simulink model "TST_PTCOP_TrqCnv"  (R2016b)
settings: Solver=FixedStepDiscrete  StartTime=0.0  StopTime=simTime  FixedStep=sampleTime  RelTol=1e-3
values from neighbouring files (symbols this model uses):
  testCase = 1    [initTST_PTCOP_TrqCnv_001.m]
libraries: simulink x8, UnitTest_Lib x6
settings Model: Creator=zhengjinyan  LastModifiedBy=zhengjinyan
settings DebuggingCC: SignalRangeChecking=error

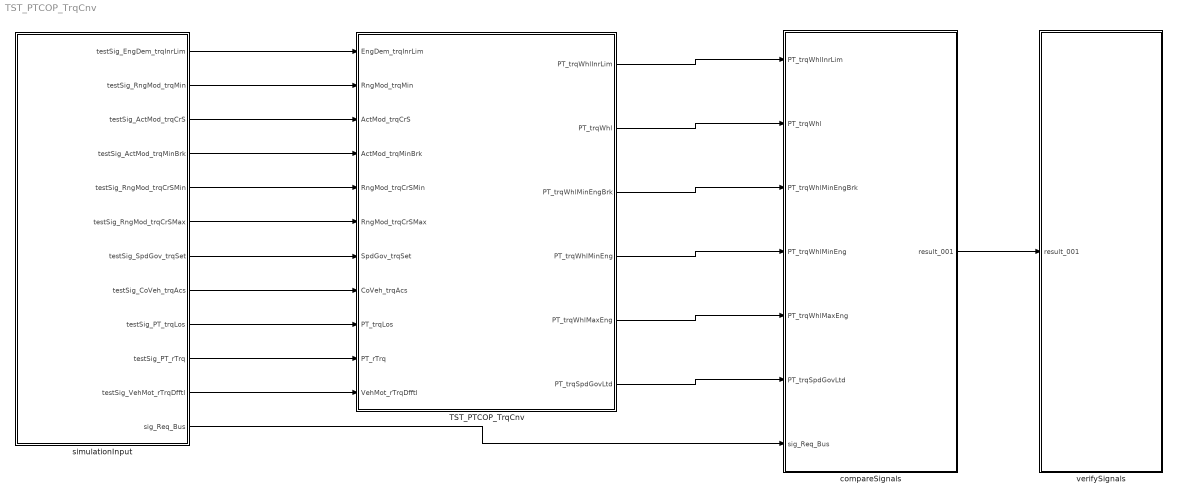
== system TST_PTCOP_TrqCnv ==
  TST_PTCOP_TrqCnv : Subsystem
  compareSignals : Subsystem
  simulationInput : Subsystem
  verifySignals : Subsystem
  wires:
  simulationInput/1(testSig_EngDem_trqInrLim) -> TST_PTCOP_TrqCnv/1(EngDem_trqInrLim)
  simulationInput/2(testSig_RngMod_trqMin) -> TST_PTCOP_TrqCnv/2(RngMod_trqMin)
  simulationInput/3(testSig_ActMod_trqCrS) -> TST_PTCOP_TrqCnv/3(ActMod_trqCrS)
  simulationInput/4(testSig_ActMod_trqMinBrk) -> TST_PTCOP_TrqCnv/4(ActMod_trqMinBrk)
  simulationInput/5(testSig_RngMod_trqCrSMin) -> TST_PTCOP_TrqCnv/5(RngMod_trqCrSMin)
  simulationInput/6(testSig_RngMod_trqCrSMax) -> TST_PTCOP_TrqCnv/6(RngMod_trqCrSMax)
  simulationInput/7(testSig_SpdGov_trqSet) -> TST_PTCOP_TrqCnv/7(SpdGov_trqSet)
  simulationInput/8(testSig_CoVeh_trqAcs) -> TST_PTCOP_TrqCnv/8(CoVeh_trqAcs)
  simulationInput/9(testSig_PT_trqLos) -> TST_PTCOP_TrqCnv/9(PT_trqLos)
  simulationInput/10(testSig_PT_rTrq) -> TST_PTCOP_TrqCnv/10(PT_rTrq)
  simulationInput/11(testSig_VehMot_rTrqDfftl) -> TST_PTCOP_TrqCnv/11(VehMot_rTrqDfftl)
  TST_PTCOP_TrqCnv/1(PT_trqWhlInrLim) -> compareSignals/1(PT_trqWhlInrLim)
  TST_PTCOP_TrqCnv/2(PT_trqWhl) -> compareSignals/2(PT_trqWhl)
  TST_PTCOP_TrqCnv/3(PT_trqWhlMinEngBrk) -> compareSignals/3(PT_trqWhlMinEngBrk)
  TST_PTCOP_TrqCnv/4(PT_trqWhlMinEng) -> compareSignals/4(PT_trqWhlMinEng)
  TST_PTCOP_TrqCnv/5(PT_trqWhlMaxEng) -> compareSignals/5(PT_trqWhlMaxEng)
  TST_PTCOP_TrqCnv/6(PT_trqSpdGovLtd) -> compareSignals/6(PT_trqSpdGovLtd)
  simulationInput/12(sig_Req_Bus) -> compareSignals/7(sig_Req_Bus)
  compareSignals/1(result_001) -> verifySignals/1(result_001)

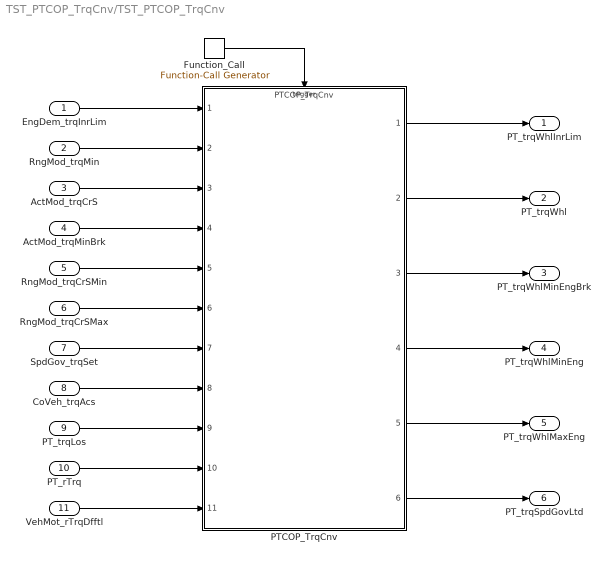
== system TST_PTCOP_TrqCnv/TST_PTCOP_TrqCnv ==
  EngDem_trqInrLim : Inport
  RngMod_trqMin : Inport  Port=2
  ActMod_trqCrS : Inport  Port=3
  ActMod_trqMinBrk : Inport  Port=4
  RngMod_trqCrSMin : Inport  Port=5
  RngMod_trqCrSMax : Inport  Port=6
  SpdGov_trqSet : Inport  Port=7
  CoVeh_trqAcs : Inport  Port=8
  PT_trqLos : Inport  Port=9
  PT_rTrq : Inport  Port=10
  VehMot_rTrqDfftl : Inport  Port=11
  Function_Call : simulink/Ports & Subsystems/Function-Call Generator  sample_time=sampleTime  numberOfIterations=1
  PTCOP_TrqCnv : ModelReference  ModelNameDialog=PTCOP_TrqCnv  SimulationMode=Normal  ModelReferenceVersion=1.5  TriggerPortName=function  TriggerPortTriggerType=function-call  TriggerPortStatesWhenEnabling=held
  PT_trqWhlInrLim : Outport
  PT_trqWhl : Outport  Port=2
  PT_trqWhlMinEngBrk : Outport  Port=3
  PT_trqWhlMinEng : Outport  Port=4
  PT_trqWhlMaxEng : Outport  Port=5
  PT_trqSpdGovLtd : Outport  Port=6
  wires:
  Function_Call/1 -> PTCOP_TrqCnv/Trigger
  EngDem_trqInrLim/1 -> PTCOP_TrqCnv/1
  RngMod_trqMin/1 -> PTCOP_TrqCnv/2
  ActMod_trqCrS/1 -> PTCOP_TrqCnv/3
  ActMod_trqMinBrk/1 -> PTCOP_TrqCnv/4
  RngMod_trqCrSMin/1 -> PTCOP_TrqCnv/5
  RngMod_trqCrSMax/1 -> PTCOP_TrqCnv/6
  SpdGov_trqSet/1 -> PTCOP_TrqCnv/7
  CoVeh_trqAcs/1 -> PTCOP_TrqCnv/8
  PT_trqLos/1 -> PTCOP_TrqCnv/9
  PT_rTrq/1 -> PTCOP_TrqCnv/10
  VehMot_rTrqDfftl/1 -> PTCOP_TrqCnv/11
  PTCOP_TrqCnv/1 -> PT_trqWhlInrLim/1
  PTCOP_TrqCnv/2 -> PT_trqWhl/1
  PTCOP_TrqCnv/3 -> PT_trqWhlMinEngBrk/1
  PTCOP_TrqCnv/4 -> PT_trqWhlMinEng/1
  PTCOP_TrqCnv/5 -> PT_trqWhlMaxEng/1
  PTCOP_TrqCnv/6 -> PT_trqSpdGovLtd/1

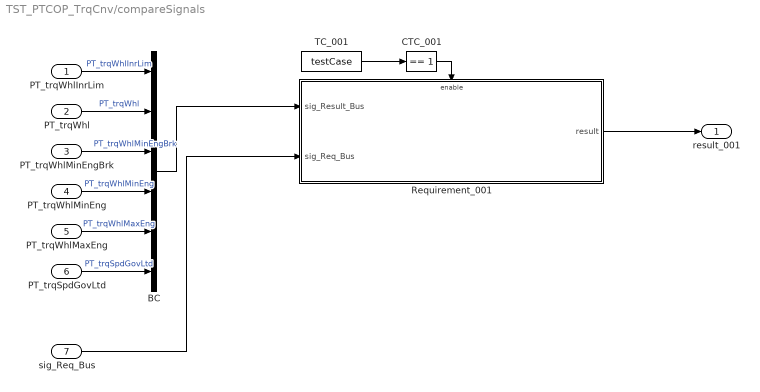
== system TST_PTCOP_TrqCnv/compareSignals ==
  PT_trqWhlInrLim : Inport
  PT_trqWhl : Inport  Port=2
  PT_trqWhlMinEngBrk : Inport  Port=3
  PT_trqWhlMinEng : Inport  Port=4
  PT_trqWhlMaxEng : Inport  Port=5
  PT_trqSpdGovLtd : Inport  Port=6
  sig_Req_Bus : Inport  Port=7
  BC : BusCreator  Inputs=6
  CTC_001 : simulink/Logic and Bit Operations/Compare To Constant  relop===  const=1  OutDataTypeStr=boolean
  Requirement_001 : Subsystem
  TC_001 : Constant  Value=testCase
  result_001 : Outport
  wires:
  PT_trqWhlInrLim/1 -> BC/1  "PT_trqWhlInrLim"
  PT_trqWhl/1 -> BC/2  "PT_trqWhl"
  PT_trqWhlMinEngBrk/1 -> BC/3  "PT_trqWhlMinEngBrk"
  PT_trqWhlMinEng/1 -> BC/4  "PT_trqWhlMinEng"
  PT_trqWhlMaxEng/1 -> BC/5  "PT_trqWhlMaxEng"
  PT_trqSpdGovLtd/1 -> BC/6  "PT_trqSpdGovLtd"
  TC_001/1 -> CTC_001/1
  CTC_001/1 -> Requirement_001/Enable
  sig_Req_Bus/1 -> Requirement_001/2(sig_Req_Bus)
  BC/1 -> Requirement_001/1(sig_Result_Bus)
  Requirement_001/1(result) -> result_001/1

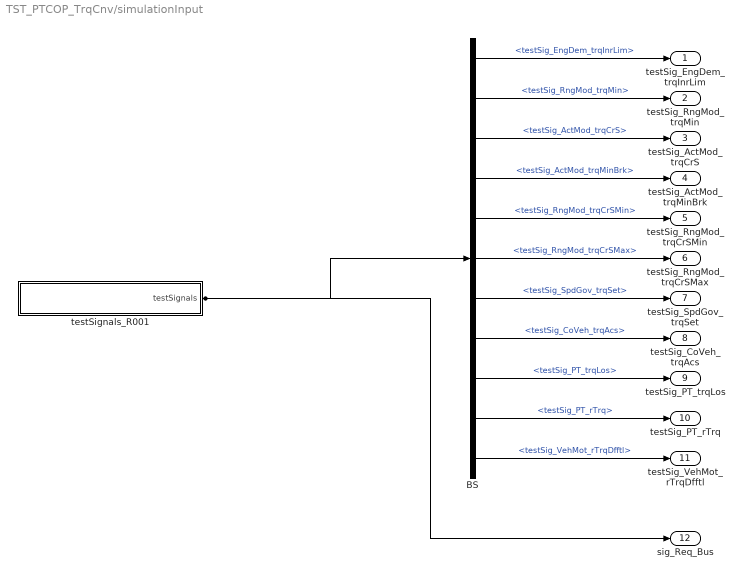
== system TST_PTCOP_TrqCnv/simulationInput ==
  BS : BusSelector  OutputSignals=testSig_EngDem_trqInrLim,testSig_RngMod_trqMin,testSig_ActMod_trqCrS,testSig_ActMod_trqMinBrk,testSig_RngMod_trqCrSMin,testSig_RngMod_trqCrSMax,testSig_SpdGov_trqSet,testSig_CoVeh_trqAcs,testSig_PT_trqLos,testSig_PT_rTrq,testSig_VehMot_rTrqDfftl
  testSignals_R001 : Subsystem
  testSig_EngDem_trqInrLim : Outport
  testSig_RngMod_trqMin : Outport  Port=2
  testSig_ActMod_trqCrS : Outport  Port=3
  testSig_ActMod_trqMinBrk : Outport  Port=4
  testSig_RngMod_trqCrSMin : Outport  Port=5
  testSig_RngMod_trqCrSMax : Outport  Port=6
  testSig_SpdGov_trqSet : Outport  Port=7
  testSig_CoVeh_trqAcs : Outport  Port=8
  testSig_PT_trqLos : Outport  Port=9
  testSig_PT_rTrq : Outport  Port=10
  testSig_VehMot_rTrqDfftl : Outport  Port=11
  sig_Req_Bus : Outport  Port=12
  wires:
  BS/1 -> testSig_EngDem_trqInrLim/1  "<testSig_EngDem_trqInrLim>"
  BS/2 -> testSig_RngMod_trqMin/1  "<testSig_RngMod_trqMin>"
  BS/3 -> testSig_ActMod_trqCrS/1  "<testSig_ActMod_trqCrS>"
  BS/4 -> testSig_ActMod_trqMinBrk/1  "<testSig_ActMod_trqMinBrk>"
  BS/5 -> testSig_RngMod_trqCrSMin/1  "<testSig_RngMod_trqCrSMin>"
  BS/6 -> testSig_RngMod_trqCrSMax/1  "<testSig_RngMod_trqCrSMax>"
  BS/7 -> testSig_SpdGov_trqSet/1  "<testSig_SpdGov_trqSet>"
  BS/8 -> testSig_CoVeh_trqAcs/1  "<testSig_CoVeh_trqAcs>"
  BS/9 -> testSig_PT_trqLos/1  "<testSig_PT_trqLos>"
  BS/10 -> testSig_PT_rTrq/1  "<testSig_PT_rTrq>"
  BS/11 -> testSig_VehMot_rTrqDfftl/1  "<testSig_VehMot_rTrqDfftl>"
  testSignals_R001/1(testSignals) -> BS/1, sig_Req_Bus/1

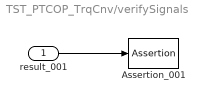
== system TST_PTCOP_TrqCnv/verifySignals ==
  result_001 : Inport
  Assertion_001 : Assertion  Enabled=off
  wires:
  result_001/1 -> Assertion_001/1

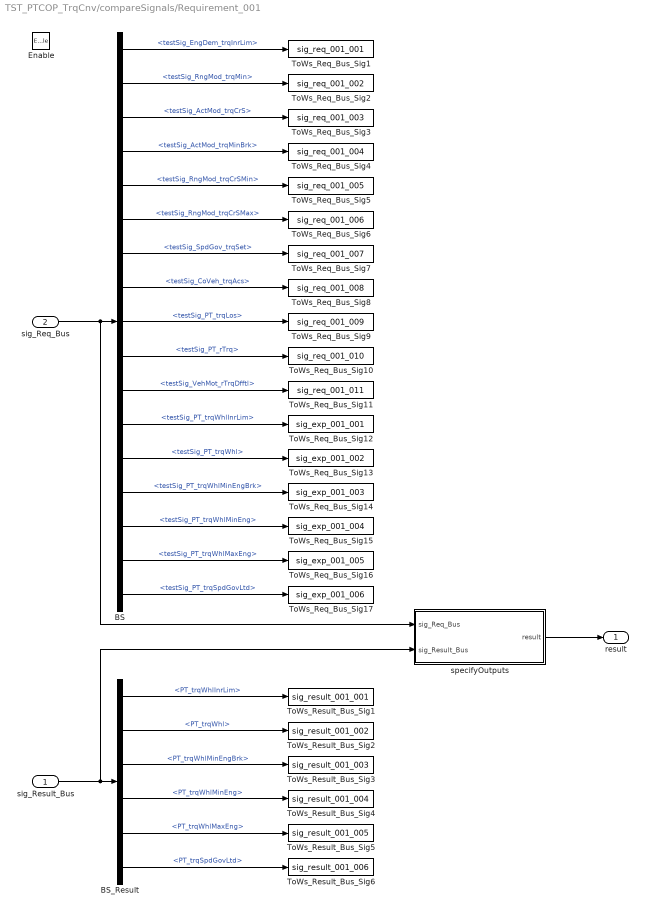
== system TST_PTCOP_TrqCnv/compareSignals/Requirement_001 ==
  sig_Result_Bus : Inport
  sig_Req_Bus : Inport  Port=2
  Enable : EnablePort
  BS : BusSelector  OutputSignals=testSig_EngDem_trqInrLim,testSig_RngMod_trqMin,testSig_ActMod_trqCrS,testSig_ActMod_trqMinBrk,testSig_RngMod_trqCrSMin,testSig_RngMod_trqCrSMax,testSig_SpdGov_trqSet,testSig_CoVeh_trqAcs,testSig_PT_trqLos,testSig_PT_rTrq,testSig_VehMot_rTrqDfftl,testSig_PT_trqWhlInrLim,testSig_PT_trqWhl,testSig_PT_trqWhlMinEngBrk,testSig_PT_trqWhlMinEng,testSig_PT_trqWhlMaxEng,testSig_PT_trqSpdGovLtd
  BS_Result : BusSelector  OutputSignals=PT_trqWhlInrLim,PT_trqWhl,PT_trqWhlMinEngBrk,PT_trqWhlMinEng,PT_trqWhlMaxEng,PT_trqSpdGovLtd
  ToWs_Req_Bus_Sig1 : ToWorkspace  VariableName=sig_req_001_001  SaveFormat=Structure With Time
  ToWs_Req_Bus_Sig10 : ToWorkspace  VariableName=sig_req_001_010  SaveFormat=Structure With Time
  ToWs_Req_Bus_Sig11 : ToWorkspace  VariableName=sig_req_001_011  SaveFormat=Structure With Time
  ToWs_Req_Bus_Sig12 : ToWorkspace  VariableName=sig_exp_001_001  SaveFormat=Structure With Time
  ToWs_Req_Bus_Sig13 : ToWorkspace  VariableName=sig_exp_001_002  SaveFormat=Structure With Time
  ToWs_Req_Bus_Sig14 : ToWorkspace  VariableName=sig_exp_001_003  SaveFormat=Structure With Time
  ToWs_Req_Bus_Sig15 : ToWorkspace  VariableName=sig_exp_001_004  SaveFormat=Structure With Time
  ToWs_Req_Bus_Sig16 : ToWorkspace  VariableName=sig_exp_001_005  SaveFormat=Structure With Time
  ToWs_Req_Bus_Sig17 : ToWorkspace  VariableName=sig_exp_001_006  SaveFormat=Structure With Time
  ToWs_Req_Bus_Sig2 : ToWorkspace  VariableName=sig_req_001_002  SaveFormat=Structure With Time
  ToWs_Req_Bus_Sig3 : ToWorkspace  VariableName=sig_req_001_003  SaveFormat=Structure With Time
  ToWs_Req_Bus_Sig4 : ToWorkspace  VariableName=sig_req_001_004  SaveFormat=Structure With Time
  ToWs_Req_Bus_Sig5 : ToWorkspace  VariableName=sig_req_001_005  SaveFormat=Structure With Time
  ToWs_Req_Bus_Sig6 : ToWorkspace  VariableName=sig_req_001_006  SaveFormat=Structure With Time
  ToWs_Req_Bus_Sig7 : ToWorkspace  VariableName=sig_req_001_007  SaveFormat=Structure With Time
  ToWs_Req_Bus_Sig8 : ToWorkspace  VariableName=sig_req_001_008  SaveFormat=Structure With Time
  ToWs_Req_Bus_Sig9 : ToWorkspace  VariableName=sig_req_001_009  SaveFormat=Structure With Time
  ToWs_Result_Bus_Sig1 : ToWorkspace  VariableName=sig_result_001_001  SaveFormat=Structure With Time
  ToWs_Result_Bus_Sig2 : ToWorkspace  VariableName=sig_result_001_002  SaveFormat=Structure With Time
  ToWs_Result_Bus_Sig3 : ToWorkspace  VariableName=sig_result_001_003  SaveFormat=Structure With Time
  ToWs_Result_Bus_Sig4 : ToWorkspace  VariableName=sig_result_001_004  SaveFormat=Structure With Time
  ToWs_Result_Bus_Sig5 : ToWorkspace  VariableName=sig_result_001_005  SaveFormat=Structure With Time
  ToWs_Result_Bus_Sig6 : ToWorkspace  VariableName=sig_result_001_006  SaveFormat=Structure With Time
  specifyOutputs : Subsystem
  result : Outport
  wires:
  sig_Req_Bus/1 -> BS/1, specifyOutputs/1(sig_Req_Bus)
  BS/1 -> ToWs_Req_Bus_Sig1/1  "<testSig_EngDem_trqInrLim>"
  BS/2 -> ToWs_Req_Bus_Sig2/1  "<testSig_RngMod_trqMin>"
  BS/3 -> ToWs_Req_Bus_Sig3/1  "<testSig_ActMod_trqCrS>"
  BS/4 -> ToWs_Req_Bus_Sig4/1  "<testSig_ActMod_trqMinBrk>"
  BS/5 -> ToWs_Req_Bus_Sig5/1  "<testSig_RngMod_trqCrSMin>"
  BS/6 -> ToWs_Req_Bus_Sig6/1  "<testSig_RngMod_trqCrSMax>"
  BS/7 -> ToWs_Req_Bus_Sig7/1  "<testSig_SpdGov_trqSet>"
  BS/8 -> ToWs_Req_Bus_Sig8/1  "<testSig_CoVeh_trqAcs>"
  BS/9 -> ToWs_Req_Bus_Sig9/1  "<testSig_PT_trqLos>"
  BS/10 -> ToWs_Req_Bus_Sig10/1  "<testSig_PT_rTrq>"
  BS/11 -> ToWs_Req_Bus_Sig11/1  "<testSig_VehMot_rTrqDfftl>"
  BS/12 -> ToWs_Req_Bus_Sig12/1  "<testSig_PT_trqWhlInrLim>"
  BS/13 -> ToWs_Req_Bus_Sig13/1  "<testSig_PT_trqWhl>"
  BS/14 -> ToWs_Req_Bus_Sig14/1  "<testSig_PT_trqWhlMinEngBrk>"
  BS/15 -> ToWs_Req_Bus_Sig15/1  "<testSig_PT_trqWhlMinEng>"
  BS/16 -> ToWs_Req_Bus_Sig16/1  "<testSig_PT_trqWhlMaxEng>"
  BS/17 -> ToWs_Req_Bus_Sig17/1  "<testSig_PT_trqSpdGovLtd>"
  sig_Result_Bus/1 -> BS_Result/1, specifyOutputs/2(sig_Result_Bus)
  BS_Result/1 -> ToWs_Result_Bus_Sig1/1  "<PT_trqWhlInrLim>"
  BS_Result/2 -> ToWs_Result_Bus_Sig2/1  "<PT_trqWhl>"
  BS_Result/3 -> ToWs_Result_Bus_Sig3/1  "<PT_trqWhlMinEngBrk>"
  BS_Result/4 -> ToWs_Result_Bus_Sig4/1  "<PT_trqWhlMinEng>"
  BS_Result/5 -> ToWs_Result_Bus_Sig5/1  "<PT_trqWhlMaxEng>"
  BS_Result/6 -> ToWs_Result_Bus_Sig6/1  "<PT_trqSpdGovLtd>"
  specifyOutputs/1(result) -> result/1

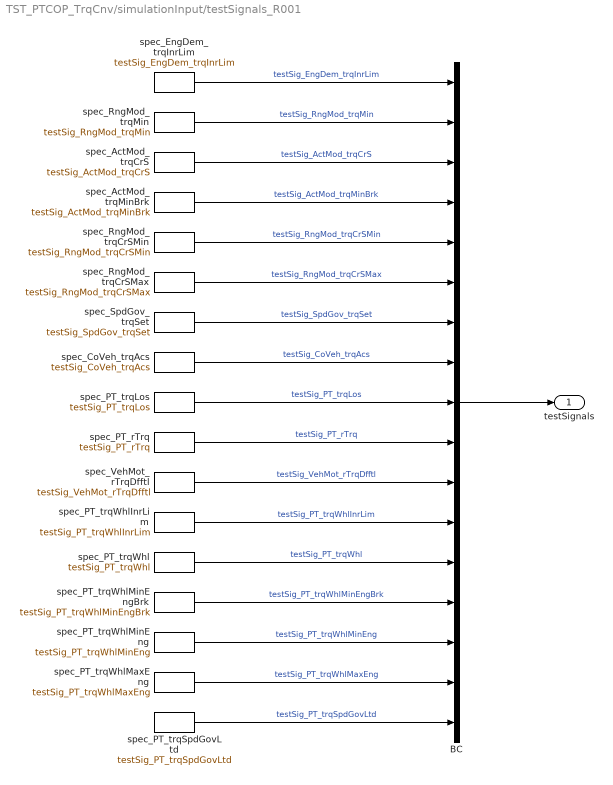
== system TST_PTCOP_TrqCnv/simulationInput/testSignals_R001 ==
  BC : BusCreator  Inputs=17
  spec_ActMod_trqCrS : FromWorkspace  VariableName=testSig_ActMod_trqCrS  Interpolate=off  OutputAfterFinalValue=Holding final value
  spec_ActMod_trqMinBrk : FromWorkspace  VariableName=testSig_ActMod_trqMinBrk  Interpolate=off  OutputAfterFinalValue=Holding final value
  spec_CoVeh_trqAcs : FromWorkspace  VariableName=testSig_CoVeh_trqAcs  Interpolate=off  OutputAfterFinalValue=Holding final value
  spec_EngDem_trqInrLim : FromWorkspace  VariableName=testSig_EngDem_trqInrLim  Interpolate=off  OutputAfterFinalValue=Holding final value
  spec_PT_rTrq : FromWorkspace  VariableName=testSig_PT_rTrq  Interpolate=off  OutputAfterFinalValue=Holding final value
  spec_PT_trqLos : FromWorkspace  VariableName=testSig_PT_trqLos  Interpolate=off  OutputAfterFinalValue=Holding final value
  spec_PT_trqSpdGovLtd : FromWorkspace  VariableName=testSig_PT_trqSpdGovLtd  Interpolate=off  OutputAfterFinalValue=Holding final value
  spec_PT_trqWhl : FromWorkspace  VariableName=testSig_PT_trqWhl  Interpolate=off  OutputAfterFinalValue=Holding final value
  spec_PT_trqWhlInrLim : FromWorkspace  VariableName=testSig_PT_trqWhlInrLim  Interpolate=off  OutputAfterFinalValue=Holding final value
  spec_PT_trqWhlMaxEng : FromWorkspace  VariableName=testSig_PT_trqWhlMaxEng  Interpolate=off  OutputAfterFinalValue=Holding final value
  spec_PT_trqWhlMinEng : FromWorkspace  VariableName=testSig_PT_trqWhlMinEng  Interpolate=off  OutputAfterFinalValue=Holding final value
  spec_PT_trqWhlMinEngBrk : FromWorkspace  VariableName=testSig_PT_trqWhlMinEngBrk  Interpolate=off  OutputAfterFinalValue=Holding final value
  spec_RngMod_trqCrSMax : FromWorkspace  VariableName=testSig_RngMod_trqCrSMax  Interpolate=off  OutputAfterFinalValue=Holding final value
  spec_RngMod_trqCrSMin : FromWorkspace  VariableName=testSig_RngMod_trqCrSMin  Interpolate=off  OutputAfterFinalValue=Holding final value
  spec_RngMod_trqMin : FromWorkspace  VariableName=testSig_RngMod_trqMin  Interpolate=off  OutputAfterFinalValue=Holding final value
  spec_SpdGov_trqSet : FromWorkspace  VariableName=testSig_SpdGov_trqSet  Interpolate=off  OutputAfterFinalValue=Holding final value
  spec_VehMot_rTrqDfftl : FromWorkspace  VariableName=testSig_VehMot_rTrqDfftl  Interpolate=off  OutputAfterFinalValue=Holding final value
  testSignals : Outport
  wires:
  BC/1 -> testSignals/1
  spec_EngDem_trqInrLim/1 -> BC/1  "testSig_EngDem_trqInrLim"
  spec_RngMod_trqMin/1 -> BC/2  "testSig_RngMod_trqMin"
  spec_ActMod_trqCrS/1 -> BC/3  "testSig_ActMod_trqCrS"
  spec_ActMod_trqMinBrk/1 -> BC/4  "testSig_ActMod_trqMinBrk"
  spec_RngMod_trqCrSMin/1 -> BC/5  "testSig_RngMod_trqCrSMin"
  spec_RngMod_trqCrSMax/1 -> BC/6  "testSig_RngMod_trqCrSMax"
  spec_SpdGov_trqSet/1 -> BC/7  "testSig_SpdGov_trqSet"
  spec_CoVeh_trqAcs/1 -> BC/8  "testSig_CoVeh_trqAcs"
  spec_PT_trqLos/1 -> BC/9  "testSig_PT_trqLos"
  spec_PT_rTrq/1 -> BC/10  "testSig_PT_rTrq"
  spec_VehMot_rTrqDfftl/1 -> BC/11  "testSig_VehMot_rTrqDfftl"
  spec_PT_trqWhlInrLim/1 -> BC/12  "testSig_PT_trqWhlInrLim"
  spec_PT_trqWhl/1 -> BC/13  "testSig_PT_trqWhl"
  spec_PT_trqWhlMinEngBrk/1 -> BC/14  "testSig_PT_trqWhlMinEngBrk"
  spec_PT_trqWhlMinEng/1 -> BC/15  "testSig_PT_trqWhlMinEng"
  spec_PT_trqWhlMaxEng/1 -> BC/16  "testSig_PT_trqWhlMaxEng"
  spec_PT_trqSpdGovLtd/1 -> BC/17  "testSig_PT_trqSpdGovLtd"

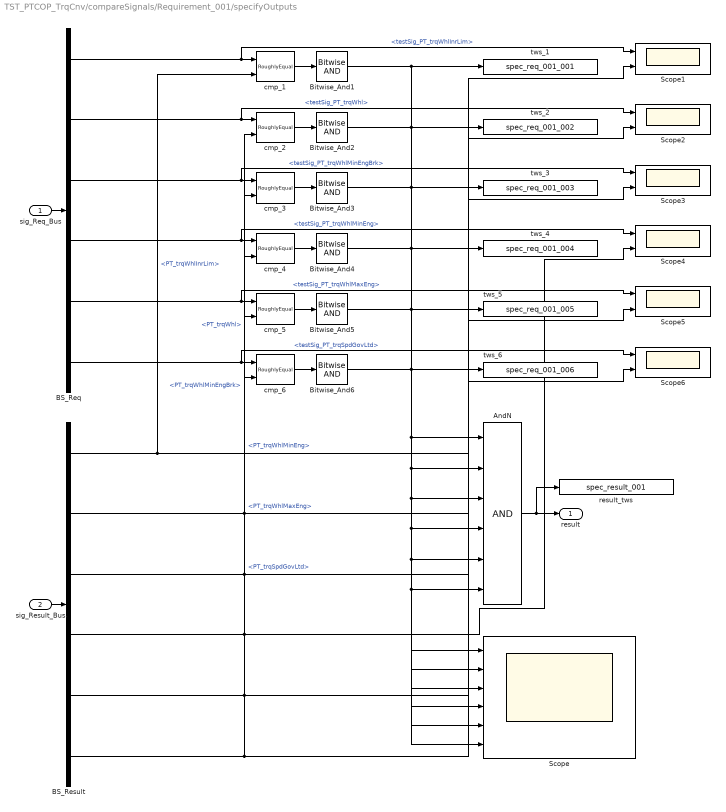
== system TST_PTCOP_TrqCnv/compareSignals/Requirement_001/specifyOutputs ==
  sig_Req_Bus : Inport
  sig_Result_Bus : Inport  Port=2
  AndN : Logic  Inputs=6
  BS_Req : BusSelector  OutputSignals=testSig_PT_trqWhlInrLim,testSig_PT_trqWhl,testSig_PT_trqWhlMinEngBrk,testSig_PT_trqWhlMinEng,testSig_PT_trqWhlMaxEng,testSig_PT_trqSpdGovLtd
  BS_Result : BusSelector  OutputSignals=PT_trqWhlInrLim,PT_trqWhl,PT_trqWhlMinEngBrk,PT_trqWhlMinEng,PT_trqWhlMaxEng,PT_trqSpdGovLtd
  Bitwise_And{1..6} (6 alike) : simulink/Logic and Bit Operations/Bitwise Operator  logicop=AND  UseBitMask=off  BitMask=bin2dec('11011001')  BitMaskRealWorld=Stored Integer
  Scope : Scope  NumInputPorts=6
  Scope{1..6} (6 alike) : Scope  NumInputPorts=2
  cmp_{1..6} (6 alike) : UnitTest_Lib/RoughlyEqual  slope=2
  result_tws : ToWorkspace  VariableName=spec_result_001
  tws_1 : ToWorkspace  VariableName=spec_req_001_001
  tws_2 : ToWorkspace  VariableName=spec_req_001_002
  tws_3 : ToWorkspace  VariableName=spec_req_001_003
  tws_4 : ToWorkspace  VariableName=spec_req_001_004
  tws_5 : ToWorkspace  VariableName=spec_req_001_005
  tws_6 : ToWorkspace  VariableName=spec_req_001_006
  result : Outport
  wires:
  sig_Req_Bus/1 -> BS_Req/1
  sig_Result_Bus/1 -> BS_Result/1
  AndN/1 -> result/1, result_tws/1
  BS_Req/1 -> cmp_1/1, Scope1/1  "<testSig_PT_trqWhlInrLim>"
  BS_Result/1 -> cmp_1/2, Scope1/2  "<PT_trqWhlInrLim>"
  cmp_1/1 -> Bitwise_And1/1
  Bitwise_And1/1 -> AndN/1, Scope/1, tws_1/1
  BS_Req/2 -> cmp_2/1, Scope2/1  "<testSig_PT_trqWhl>"
  BS_Result/2 -> cmp_2/2, Scope2/2  "<PT_trqWhl>"
  cmp_2/1 -> Bitwise_And2/1
  Bitwise_And2/1 -> AndN/2, Scope/2, tws_2/1
  BS_Req/3 -> cmp_3/1, Scope3/1  "<testSig_PT_trqWhlMinEngBrk>"
  BS_Result/3 -> cmp_3/2, Scope3/2  "<PT_trqWhlMinEngBrk>"
  cmp_3/1 -> Bitwise_And3/1
  Bitwise_And3/1 -> AndN/3, Scope/3, tws_3/1
  BS_Req/4 -> cmp_4/1, Scope4/1  "<testSig_PT_trqWhlMinEng>"
  BS_Result/4 -> cmp_4/2, Scope4/2  "<PT_trqWhlMinEng>"
  cmp_4/1 -> Bitwise_And4/1
  Bitwise_And4/1 -> AndN/4, Scope/4, tws_4/1
  BS_Req/5 -> cmp_5/1, Scope5/1  "<testSig_PT_trqWhlMaxEng>"
  BS_Result/5 -> cmp_5/2, Scope5/2  "<PT_trqWhlMaxEng>"
  cmp_5/1 -> Bitwise_And5/1
  Bitwise_And5/1 -> AndN/5, Scope/5, tws_5/1
  BS_Req/6 -> cmp_6/1, Scope6/1  "<testSig_PT_trqSpdGovLtd>"
  BS_Result/6 -> cmp_6/2, Scope6/2  "<PT_trqSpdGovLtd>"
  cmp_6/1 -> Bitwise_And6/1
  Bitwise_And6/1 -> AndN/6, Scope/6, tws_6/1
